simulink model "simulation_upgrade"  (R2024b)
settings: Solver=ode1be  StartTime=0.0  StopTime=10  FixedStep=0.001  RelTol=1e-3
model workspace (MAT data in the model file):
  AMP = 1
  FREQ = 1
  i_abc = 1
values from neighbouring files (symbols this model uses):
  v_WLTP = [0 0 0 0 0 0 0 0 0 0 0 0 ... (180001 elements, 1x180001)]    [v_WLTP.mat]
undefined symbols (not defined in the file or in its folder): A, a_sig, b_sig, C1, C2, C3, Cd, CG_z, downshift, Drive_wheel, Driveshaft, f_blend, f_OVD, fo, front_seat_dist, fs, g, Gearbox, i, i_sig, Inclination, Inertia, Jr2, K, m, M_curve_1, M_curve_2, m_driver, M_N_1, M_N_2, mi_c, mi_s, Mode, N_clutch, n_curve_1, n_curve_2, n_driver, n_max_1, n_max_2, n_shift, n_surfaces, Pl, Planetary, r_eq_clutch, r_geom, r_wheel, rho, Shaft, shift_time, sigma0, sigma1, sigma2, slope_angle, Stage1, Stage2, Stage3, upshift, v0, vel_wind, vs ... (+5)
libraries: simulink x29, slpidlib x3
(part 7 of 9)

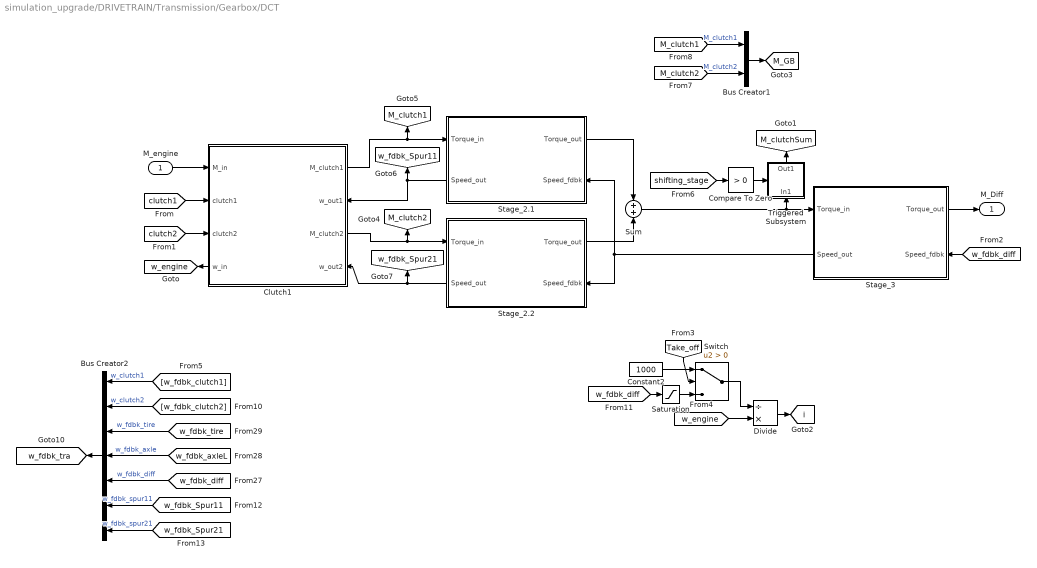
== system simulation_upgrade/DRIVETRAIN/Transmission/Gearbox/DCT ==
  M_engine : Inport
  Bus Creator1 : BusCreator  Inputs=2
  Bus Creator2 : BusCreator  Inputs=7
  Clutch1 : Subsystem
      settings: PortSchema="{\"entries\":[{\"content\":{\"sides\":[{\"content\":{\"connectorIds\":[\"In1\",\"In2\",\"In3\",\"Out3\"]},\"type\":\"ConnectorPlacement.EquallySpacedRectSide\",\"uuid\":\"d6060937-6a70-4d8f-85b8-f3c9c5d18f93\"},{\"content\":{\"connectorIds\":[\"Out1\",\"In4\",\"Out2\",\"In5\"],\"side\":\"RIGHT\"},\"type\":\"ConnectorPlacement.EquallySpacedRectSide\",\"uuid\":\"5f6b068d-fc68-4249-8013-bc3df4965ca3\"},{\"content\":{\"side\":\"TOP\"},\"type\":\"ConnectorPlacement.EquallySpacedRectSide\",\"uuid\":\"81b536de-881e-418d-8c02-7373631e1270\"}]},\"type\":\"ConnectorPlacement.EquallySpacedConnector\",\"uuid\":\"48438dfd-c2d0-4ff7-b57e-a1bd101206eb\"}],\"packageUris\":[\"http://schema.mathworks.com/mf0/Connector/R2020b\"],\"version\":\"1.0\"}"
      mask Display: image('images/clutch.jpg');
  Compare To Zero : simulink/Logic and Bit Operations/Compare To Zero  relop=>  OutDataTypeStr=boolean
  Constant2 : Constant  Value=1000
  Divide : Product  Inputs=/*
  Saturation : Saturate  UpperLimit=1000000  LowerLimit=1
  Stage_2.1 : Subsystem  Variant=on
      settings: PortSchema="{\"entries\":[{\"content\":{\"sides\":[{\"content\":{\"connectorIds\":[\"In1\",\"Out2\"]},\"type\":\"ConnectorPlacement.EquallySpacedRectSide\",\"uuid\":\"898fedf9-82f7-4bc2-bf05-880de36b191d\"},{\"content\":{\"connectorIds\":[\"Out1\",\"In2\"],\"side\":\"RIGHT\"},\"type\":\"ConnectorPlacement.EquallySpacedRectSide\",\"uuid\":\"50317b6c-245f-4bd1-a8cd-7a774957ae86\"},{\"content\":{\"side\":\"TOP\"},\"type\":\"ConnectorPlacement.EquallySpacedRectSide\",\"uuid\":\"ff1de2a1-7305-40d8-9e1f-fd0fa1e7d830\"}]},\"type\":\"ConnectorPlacement.EquallySpacedConnector\",\"uuid\":\"6ce82d73-f3da-4f59-9039-464a6ef3e9c5\"}],\"packageUris\":[\"http://schema.mathworks.com/mf0/Connector/R2020b\"],\"version\":\"1.0\"}"
      mask Display: image('images/branco.png');
  Stage_2.2 : Subsystem  Variant=on
      settings: PortSchema="{\"entries\":[{\"content\":{\"sides\":[{\"content\":{\"connectorIds\":[\"In1\",\"Out2\"]},\"type\":\"ConnectorPlacement.EquallySpacedRectSide\",\"uuid\":\"898fedf9-82f7-4bc2-bf05-880de36b191d\"},{\"content\":{\"connectorIds\":[\"Out1\",\"In2\"],\"side\":\"RIGHT\"},\"type\":\"ConnectorPlacement.EquallySpacedRectSide\",\"uuid\":\"50317b6c-245f-4bd1-a8cd-7a774957ae86\"},{\"content\":{\"side\":\"TOP\"},\"type\":\"ConnectorPlacement.EquallySpacedRectSide\",\"uuid\":\"ff1de2a1-7305-40d8-9e1f-fd0fa1e7d830\"}]},\"type\":\"ConnectorPlacement.EquallySpacedConnector\",\"uuid\":\"6ce82d73-f3da-4f59-9039-464a6ef3e9c5\"}],\"packageUris\":[\"http://schema.mathworks.com/mf0/Connector/R2020b\"],\"version\":\"1.0\"}"
      mask Display: image('images/branco.png');
  Stage_3 : Subsystem  Variant=on
      settings: PortSchema="{\"entries\":[{\"content\":{\"sides\":[{\"content\":{\"connectorIds\":[\"In1\",\"Out2\"]},\"type\":\"ConnectorPlacement.EquallySpacedRectSide\",\"uuid\":\"37b17ee8-4b62-4191-976c-22442f171034\"},{\"content\":{\"connectorIds\":[\"Out1\",\"In2\"],\"side\":\"RIGHT\"},\"type\":\"ConnectorPlacement.EquallySpacedRectSide\",\"uuid\":\"4dd88878-371f-49ed-bf90-7ed62e5325b4\"},{\"content\":{\"side\":\"TOP\"},\"type\":\"ConnectorPlacement.EquallySpacedRectSide\",\"uuid\":\"77efb153-e78e-4021-a08b-14751aa491e1\"}]},\"type\":\"ConnectorPlacement.EquallySpacedConnector\",\"uuid\":\"fa13ac12-58ae-4dfa-a455-8cf832864b15\"}],\"packageUris\":[\"http://schema.mathworks.com/mf0/Connector/R2020b\"],\"version\":\"1.0\"}"
      mask Display: image('images/branco.png');
  Sum : Sum  Inputs=+|+
  Switch : Switch  Criteria=u2 > Threshold  SaturateOnIntegerOverflow=off  InputSameDT=off
  Triggered Subsystem : Subsystem  TreatAsAtomicUnit=on
  M_Diff : Outport
  tag scope: M_GB=global, M_clutch1=global, M_clutch2=global, M_clutchSum=global, i=global, w_engine=global, w_fdbk_Spur11=global, w_fdbk_Spur21=global, w_fdbk_tra=global
  wires:
  Clutch1/1(M_clutch1) -> Stage_2.1/1(Torque_in), [M_clutch1]
  Bus Creator1/1 -> [M_GB]
  [w_fdbk_tire] -> Bus Creator2/3  "w_fdbk_tire"
  Switch/1 -> Divide/1
  [M_clutch1] -> Bus Creator1/1  "M_clutch1"
  [w_fdbk_clutch1] -> Bus Creator2/1  "w_clutch1"
  M_engine/1 -> Clutch1/1(M_in)
  Stage_3/2(Speed_out) -> Stage_2.1/2(Speed_fdbk), Stage_2.2/2(Speed_fdbk)
  [w_fdbk_diff] -> Saturation/1
  [w_fdbk_axleL] -> Bus Creator2/4  "w_fdbk_axle"
  [Take_off] -> Switch/2
  Bus Creator2/1 -> [w_fdbk_tra]
  [w_fdbk_diff] -> Stage_3/2(Speed_fdbk)
  Constant2/1 -> Switch/1
  Stage_3/1(Torque_out) -> M_Diff/1
  [w_fdbk_Spur21] -> Bus Creator2/7  "w_fdbk_spur21"
  Stage_2.1/2(Speed_out) -> Clutch1/4(w_out1), [w_fdbk_Spur11]
  Stage_2.1/1(Torque_out) -> Sum/1
  Stage_2.2/2(Speed_out) -> Clutch1/5(w_out2), [w_fdbk_Spur21]
  [w_fdbk_diff] -> Bus Creator2/5  "w_fdbk_diff"
  Divide/1 -> [i]
  Stage_2.2/1(Torque_out) -> Sum/2
  [w_fdbk_clutch2] -> Bus Creator2/2  "w_clutch2"
  [M_clutch2] -> Bus Creator1/2  "M_clutch2"
  [w_engine] -> Divide/2
  Saturation/1 -> Switch/3
  [w_fdbk_Spur11] -> Bus Creator2/6  "w_fdbk_spur11"
  Sum/1 -> Stage_3/1(Torque_in), Triggered Subsystem/1(In1)
  Clutch1/2(M_clutch2) -> [M_clutch2], Stage_2.2/1(Torque_in)
  Clutch1/3(w_in) -> [w_engine]
  [clutch1] -> Clutch1/2(clutch1)
  [clutch2] -> Clutch1/3(clutch2)
  Triggered Subsystem/1(Out1) -> [M_clutchSum]
  Compare To Zero/1 -> Triggered Subsystem/Trigger
  [shifting_stage] -> Compare To Zero/1

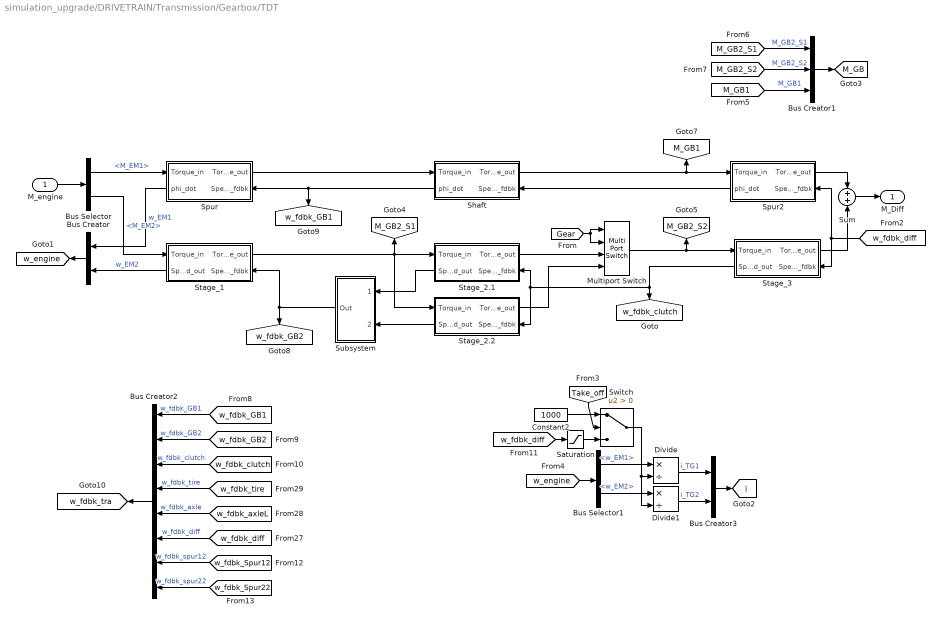
== system simulation_upgrade/DRIVETRAIN/Transmission/Gearbox/TDT ==
  M_engine : Inport
  Bus Creator : BusCreator  Inputs=2
  Bus Creator1 : BusCreator  Inputs=3
  Bus Creator2 : BusCreator  Inputs=8
  Bus Creator3 : BusCreator  Inputs=2
  Bus Selector : BusSelector  OutputSignals=M_EM1,M_EM2
  Bus Selector1 : BusSelector  OutputSignals=w_EM1,w_EM2
  Constant2 : Constant  Value=1000
  Divide : Product  Inputs=*/
  Divide1 : Product  Inputs=*/
  Multiport Switch : MultiPortSwitch  DataPortOrder=Zero-based contiguous  zeroidx=on  SaturateOnIntegerOverflow=off  InputSameDT=off
  Saturation : Saturate  UpperLimit=1000000  LowerLimit=1
  Shaft : Subsystem  mask{J=Shaft.J}
      mask prompts: J "Inertia_kgm^2"
      settings: PortSchema="{\"entries\":[{\"content\":{\"sides\":[{\"content\":{\"connectorIds\":[\"In1\",\"Out2\"]},\"type\":\"ConnectorPlacement.EquallySpacedRectSide\",\"uuid\":\"898fedf9-82f7-4bc2-bf05-880de36b191d\"},{\"content\":{\"connectorIds\":[\"Out1\",\"In2\"],\"side\":\"RIGHT\"},\"type\":\"ConnectorPlacement.EquallySpacedRectSide\",\"uuid\":\"50317b6c-245f-4bd1-a8cd-7a774957ae86\"},{\"content\":{\"side\":\"TOP\"},\"type\":\"ConnectorPlacement.EquallySpacedRectSide\",\"uuid\":\"ff1de2a1-7305-40d8-9e1f-fd0fa1e7d830\"}]},\"type\":\"ConnectorPlacement.EquallySpacedConnector\",\"uuid\":\"6ce82d73-f3da-4f59-9039-464a6ef3e9c5\"}],\"packageUris\":[\"http://schema.mathworks.com/mf0/Connector/R2020b\"],\"version\":\"1.0\"}"
  Spur : Subsystem  mask{i=Stage2.i1, J1=Stage2.Spur11.J, J2=Stage2.Spur12.J}
      mask prompts: i "Ratio"; J1 "Input_Gear_Inertia"; J2 "Output_Gear_Inertia"
      settings: PortSchema="{\"entries\":[{\"content\":{\"sides\":[{\"content\":{\"connectorIds\":[\"In1\",\"Out2\"]},\"type\":\"ConnectorPlacement.EquallySpacedRectSide\",\"uuid\":\"898fedf9-82f7-4bc2-bf05-880de36b191d\"},{\"content\":{\"connectorIds\":[\"Out1\",\"In2\"],\"side\":\"RIGHT\"},\"type\":\"ConnectorPlacement.EquallySpacedRectSide\",\"uuid\":\"50317b6c-245f-4bd1-a8cd-7a774957ae86\"},{\"content\":{\"side\":\"TOP\"},\"type\":\"ConnectorPlacement.EquallySpacedRectSide\",\"uuid\":\"ff1de2a1-7305-40d8-9e1f-fd0fa1e7d830\"}]},\"type\":\"ConnectorPlacement.EquallySpacedConnector\",\"uuid\":\"6ce82d73-f3da-4f59-9039-464a6ef3e9c5\"}],\"packageUris\":[\"http://schema.mathworks.com/mf0/Connector/R2020b\"],\"version\":\"1.0\"}"
  Spur2 : Subsystem  mask{i=Stage2.i1, J1=Stage2.Spur11.J, J2=Stage2.Spur12.J}
      mask prompts: i "Ratio"; J1 "Input_Gear_Inertia"; J2 "Output_Gear_Inertia"
      settings: PortSchema="{\"entries\":[{\"content\":{\"sides\":[{\"content\":{\"connectorIds\":[\"In1\",\"Out2\"]},\"type\":\"ConnectorPlacement.EquallySpacedRectSide\",\"uuid\":\"898fedf9-82f7-4bc2-bf05-880de36b191d\"},{\"content\":{\"connectorIds\":[\"Out1\",\"In2\"],\"side\":\"RIGHT\"},\"type\":\"ConnectorPlacement.EquallySpacedRectSide\",\"uuid\":\"50317b6c-245f-4bd1-a8cd-7a774957ae86\"},{\"content\":{\"side\":\"TOP\"},\"type\":\"ConnectorPlacement.EquallySpacedRectSide\",\"uuid\":\"ff1de2a1-7305-40d8-9e1f-fd0fa1e7d830\"}]},\"type\":\"ConnectorPlacement.EquallySpacedConnector\",\"uuid\":\"6ce82d73-f3da-4f59-9039-464a6ef3e9c5\"}],\"packageUris\":[\"http://schema.mathworks.com/mf0/Connector/R2020b\"],\"version\":\"1.0\"}"
  Stage_1 : Subsystem  Variant=on
      settings: PortSchema="{\"entries\":[{\"content\":{\"sides\":[{\"content\":{\"connectorIds\":[\"In1\",\"Out2\"]},\"type\":\"ConnectorPlacement.EquallySpacedRectSide\",\"uuid\":\"898fedf9-82f7-4bc2-bf05-880de36b191d\"},{\"content\":{\"connectorIds\":[\"Out1\",\"In2\"],\"side\":\"RIGHT\"},\"type\":\"ConnectorPlacement.EquallySpacedRectSide\",\"uuid\":\"50317b6c-245f-4bd1-a8cd-7a774957ae86\"},{\"content\":{\"side\":\"TOP\"},\"type\":\"ConnectorPlacement.EquallySpacedRectSide\",\"uuid\":\"ff1de2a1-7305-40d8-9e1f-fd0fa1e7d830\"}]},\"type\":\"ConnectorPlacement.EquallySpacedConnector\",\"uuid\":\"6ce82d73-f3da-4f59-9039-464a6ef3e9c5\"}],\"packageUris\":[\"http://schema.mathworks.com/mf0/Connector/R2020b\"],\"version\":\"1.0\"}"
      mask Display: image('images/branco.png');
  Stage_2.1 : Subsystem  Variant=on
      settings: PortSchema="{\"entries\":[{\"content\":{\"sides\":[{\"content\":{\"connectorIds\":[\"In1\",\"Out2\"]},\"type\":\"ConnectorPlacement.EquallySpacedRectSide\",\"uuid\":\"898fedf9-82f7-4bc2-bf05-880de36b191d\"},{\"content\":{\"connectorIds\":[\"Out1\",\"In2\"],\"side\":\"RIGHT\"},\"type\":\"ConnectorPlacement.EquallySpacedRectSide\",\"uuid\":\"50317b6c-245f-4bd1-a8cd-7a774957ae86\"},{\"content\":{\"side\":\"TOP\"},\"type\":\"ConnectorPlacement.EquallySpacedRectSide\",\"uuid\":\"ff1de2a1-7305-40d8-9e1f-fd0fa1e7d830\"}]},\"type\":\"ConnectorPlacement.EquallySpacedConnector\",\"uuid\":\"6ce82d73-f3da-4f59-9039-464a6ef3e9c5\"}],\"packageUris\":[\"http://schema.mathworks.com/mf0/Connector/R2020b\"],\"version\":\"1.0\"}"
      mask Display: image('images/branco.png');
  Stage_2.2 : Subsystem  Variant=on
      settings: PortSchema="{\"entries\":[{\"content\":{\"sides\":[{\"content\":{\"connectorIds\":[\"In1\",\"Out2\"]},\"type\":\"ConnectorPlacement.EquallySpacedRectSide\",\"uuid\":\"898fedf9-82f7-4bc2-bf05-880de36b191d\"},{\"content\":{\"connectorIds\":[\"Out1\",\"In2\"],\"side\":\"RIGHT\"},\"type\":\"ConnectorPlacement.EquallySpacedRectSide\",\"uuid\":\"50317b6c-245f-4bd1-a8cd-7a774957ae86\"},{\"content\":{\"side\":\"TOP\"},\"type\":\"ConnectorPlacement.EquallySpacedRectSide\",\"uuid\":\"ff1de2a1-7305-40d8-9e1f-fd0fa1e7d830\"}]},\"type\":\"ConnectorPlacement.EquallySpacedConnector\",\"uuid\":\"6ce82d73-f3da-4f59-9039-464a6ef3e9c5\"}],\"packageUris\":[\"http://schema.mathworks.com/mf0/Connector/R2020b\"],\"version\":\"1.0\"}"
      mask Display: image('images/branco.png');
  Stage_3 : Subsystem  Variant=on
      settings: PortSchema="{\"entries\":[{\"content\":{\"sides\":[{\"content\":{\"connectorIds\":[\"In1\",\"Out2\"]},\"type\":\"ConnectorPlacement.EquallySpacedRectSide\",\"uuid\":\"898fedf9-82f7-4bc2-bf05-880de36b191d\"},{\"content\":{\"connectorIds\":[\"Out1\",\"In2\"],\"side\":\"RIGHT\"},\"type\":\"ConnectorPlacement.EquallySpacedRectSide\",\"uuid\":\"50317b6c-245f-4bd1-a8cd-7a774957ae86\"},{\"content\":{\"side\":\"TOP\"},\"type\":\"ConnectorPlacement.EquallySpacedRectSide\",\"uuid\":\"ff1de2a1-7305-40d8-9e1f-fd0fa1e7d830\"}]},\"type\":\"ConnectorPlacement.EquallySpacedConnector\",\"uuid\":\"6ce82d73-f3da-4f59-9039-464a6ef3e9c5\"}],\"packageUris\":[\"http://schema.mathworks.com/mf0/Connector/R2020b\"],\"version\":\"1.0\"}"
      mask Display: image('images/branco.png');
  Subsystem : Subsystem
      settings: PortSchema="{\"entries\":[{\"content\":{\"sides\":[{\"content\":{\"connectorIds\":[\"Out1\"]},\"type\":\"ConnectorPlacement.EquallySpacedRectSide\",\"uuid\":\"fb6fb521-24b4-42a9-962b-0690c95a6555\"},{\"content\":{\"connectorIds\":[\"In1\",\"In2\"],\"side\":\"RIGHT\"},\"type\":\"ConnectorPlacement.EquallySpacedRectSide\",\"uuid\":\"05ff3728-9142-4ede-8c02-c3816594f1d6\"},{\"content\":{\"side\":\"TOP\"},\"type\":\"ConnectorPlacement.EquallySpacedRectSide\",\"uuid\":\"6bf5bb06-bb76-41b4-800b-6d1bd3df4c7c\"}]},\"type\":\"ConnectorPlacement.EquallySpacedConnector\",\"uuid\":\"4f0648fe-100b-4dfa-b2f8-0696c3f6a986\"}],\"packageUris\":[\"http://schema.mathworks.com/mf0/Connector/R2020b\"],\"version\":\"1.0\"}"
  Sum : Sum  Inputs=+|+
  Switch : Switch  Criteria=u2 > Threshold  SaturateOnIntegerOverflow=off  InputSameDT=off
  M_Diff : Outport
  tag scope: M_GB1=global, M_GB2_S1=global, M_GB2_S2=global, M_GB=global, i=global, w_engine=global, w_fdbk_GB1=global, w_fdbk_GB2=global, w_fdbk_clutch=global, w_fdbk_tra=global
  wires:
  M_engine/1 -> Bus Selector/1
  [Gear] -> Multiport Switch/2, Multiport Switch/1
  Multiport Switch/1 -> [M_GB2_S2], Stage_3/1(Torque_in)
  Stage_2.1/1(Torque_out) -> Multiport Switch/3
  Stage_1/2(Speed_out) -> Bus Creator/2  "w_EM2"
  Stage_2.2/1(Torque_out) -> Multiport Switch/4
  Stage_3/1(Torque_out) -> Sum/2
  Stage_2.1/2(Speed_out) -> Subsystem/1(Spur 21)
  Subsystem/1(Out) -> [w_fdbk_GB2], Stage_1/2(Speed_fdbk)
  Stage_3/2(Speed_out) -> Stage_2.2/2(Speed_fdbk), Stage_2.1/2(Speed_fdbk), [w_fdbk_clutch]
  Stage_1/1(Torque_out) -> Stage_2.1/1(Torque_in), [M_GB2_S1], Stage_2.2/1(Torque_in)
  Stage_2.2/2(Speed_out) -> Subsystem/2(Spur22)
  Shaft/1(Torque_out) -> Spur2/1(Torque_in), [M_GB1]
  Spur/1(Torque_out) -> Shaft/1(Torque_in)
  Spur2/2(phi_dot) -> Shaft/2(Speed_fdbk)
  Spur2/1(Torque_out) -> Sum/1
  [w_fdbk_diff] -> Spur2/2(Speed_fdbk), Stage_3/2(Speed_fdbk)
  Shaft/2(phi_dot) -> Spur/2(Speed_fdbk), [w_fdbk_GB1]
  Spur/2(phi_dot) -> Bus Creator/1  "w_EM1"
  Sum/1 -> M_Diff/1
  Bus Selector/2 -> Stage_1/1(Torque_in)  "<M_EM2>"
  Bus Selector/1 -> Spur/1(Torque_in)  "<M_EM1>"
  Bus Creator/1 -> [w_engine]
  Bus Creator1/1 -> [M_GB]
  [M_GB2_S2] -> Bus Creator1/2  "M_GB2_S2"
  [M_GB1] -> Bus Creator1/3  "M_GB1"
  [M_GB2_S1] -> Bus Creator1/1  "M_GB2_S1"
  [w_fdbk_GB1] -> Bus Creator2/1  "w_fdbk_GB1"
  [w_fdbk_GB2] -> Bus Creator2/2  "w_fdbk_GB2"
  [w_fdbk_clutch] -> Bus Creator2/3  "w_fdbk_clutch"
  Bus Creator2/1 -> [w_fdbk_tra]
  [w_fdbk_tire] -> Bus Creator2/4  "w_fdbk_tire"
  [w_fdbk_axleL] -> Bus Creator2/5  "w_fdbk_axle"
  [w_fdbk_diff] -> Bus Creator2/6  "w_fdbk_diff"
  [w_engine] -> Bus Selector1/1
  Bus Selector1/1 -> Divide/1  "<w_EM1>"
  Bus Selector1/2 -> Divide1/1  "<w_EM2>"
  Switch/1 -> Divide1/2, Divide/2
  Divide/1 -> Bus Creator3/1  "i_TG1"
  Divide1/1 -> Bus Creator3/2  "i_TG2"
  [w_fdbk_diff] -> Saturation/1
  [Take_off] -> Switch/2
  Constant2/1 -> Switch/1
  Bus Creator3/1 -> [i]
  Saturation/1 -> Switch/3
  [w_fdbk_Spur12] -> Bus Creator2/7  "w_fdbk_spur12"
  [w_fdbk_Spur22] -> Bus Creator2/8  "w_fdbk_spur22"

== system simulation_upgrade/DRIVETRAIN/Transmission/Gearbox/e-CVT ==
  M_engine : Inport
  M_Diff : Outport
  wires:
  M_engine/1 -> M_Diff/1

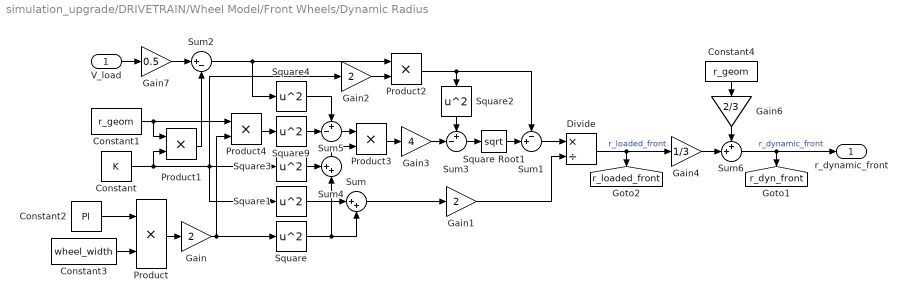
== system simulation_upgrade/DRIVETRAIN/Wheel Model/Front Wheels/Dynamic Radius ==
  V_load : Inport
  Constant : Constant  Value=K
  Constant1 : Constant  Value=r_geom
  Constant2 : Constant  Value=Pl
  Constant3 : Constant  Value=wheel_width
  Constant4 : Constant  Value=r_geom
  Divide : Product  Inputs=*/
  Gain : Gain  Gain=2
  Gain1 : Gain  Gain=2
  Gain2 : Gain  Gain=2
  Gain3 : Gain  Gain=4
  Gain4 : Gain  Gain=1/3
  Gain6 : Gain  Gain=2/3
  Gain7 : Gain  Gain=0.5
  Product{,1..4} (5 alike) : Product
  Square{,1..4,9} (6 alike) : Math  Operator=square
  Square Root1 : Sqrt
  Sum : Sum  Inputs=|++
  Sum1 : Sum  Inputs=-+|
  Sum2 : Sum  Inputs=|+-
  Sum3 : Sum  Inputs=+-|
  Sum4 : Sum  Inputs=++|
  Sum5 : Sum  Inputs=+-|
  Sum6 : Sum  Inputs=++|
  r_dynamic_front : Outport
  tag scope: r_dyn_front=global, r_loaded_front=global
  wires:
  Square1/1 -> Sum/1
  Divide/1 -> Gain4/1, [r_loaded_front]  "r_loaded_front"
  Square3/1 -> Sum4/1
  Sum/1 -> Gain1/1
  Sum1/1 -> Divide/1
  Constant/1 -> Product1/2, Square3/1, Gain2/1, Square1/1
  Constant3/1 -> Product/2
  Product1/1 -> Sum2/2
  Square Root1/1 -> Sum1/2
  Gain3/1 -> Sum3/2
  Gain/1 -> Product4/2, Square/1
  Constant2/1 -> Product/1
  Sum5/1 -> Product3/1
  Product3/1 -> Gain3/1
  Gain1/1 -> Divide/2
  Constant1/1 -> Product4/1, Product1/1
  Square9/1 -> Sum5/2
  Square/1 -> Sum4/2, Sum/2
  Sum4/1 -> Product3/2
  Sum3/1 -> Square Root1/1
  Square4/1 -> Sum5/1
  Sum2/1 -> Square4/1, Product2/1
  Product4/1 -> Square9/1
  Product/1 -> Gain/1
  Square2/1 -> Sum3/1
  Gain4/1 -> Sum6/2
  Gain6/1 -> Sum6/1
  Gain7/1 -> Sum2/1
  Constant4/1 -> Gain6/1
  Gain2/1 -> Product2/2
  Sum6/1 -> r_dynamic_front/1, [r_dyn_front]  "r_dynamic_front"
  Product2/1 -> Square2/1, Sum1/1
  V_load/1 -> Gain7/1

== system simulation_upgrade/DRIVETRAIN/Wheel Model/Front Wheels/Wheel Torque ==
  M_tra : Inport
  M_break : Inport  Port=2
  Bus Selector1 : BusSelector  OutputSignals=M_axleL,M_axleR
  Constant5 : Constant  Value=Drive_wheel
  Gain9 : Gain  Gain=0.5
  Multiport Switch : MultiPortSwitch  DataPortOrder=Zero-based contiguous  zeroidx=on  SaturateOnIntegerOverflow=off  InputSameDT=off
  Sum3 : Sum  Inputs=++|
  Sum4 : Sum  Inputs=++|
  Sum8 : Sum  Inputs=+|+
  M_front_wheels : Outport
  tag scope: M_front_wheels=global
  wires:
  Multiport Switch/1 -> M_front_wheels/1, [M_front_wheels]  "M_front_wheels"
  Bus Selector1/1 -> Sum8/1  "<M_axleL>"
  Constant5/1 -> Multiport Switch/1
  Gain9/1 -> Sum3/2
  M_break/1 -> Sum4/1, Sum3/1, Multiport Switch/2
  Bus Selector1/2 -> Sum8/2  "<M_axleR>"
  M_tra/1 -> Bus Selector1/1
  Sum8/1 -> Sum4/2, Gain9/1
  Sum3/1 -> Multiport Switch/4
  Sum4/1 -> Multiport Switch/3

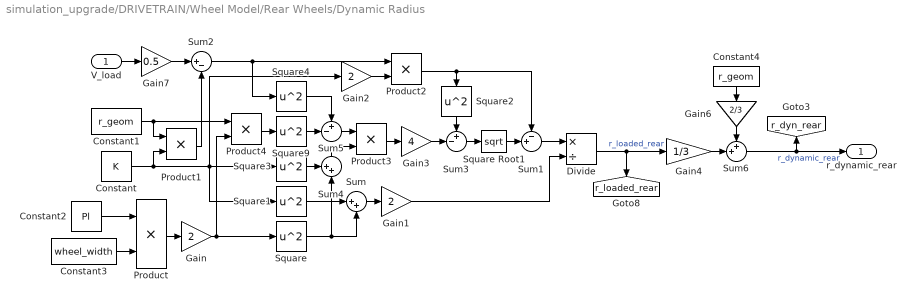
== system simulation_upgrade/DRIVETRAIN/Wheel Model/Rear Wheels/Dynamic Radius ==
  V_load : Inport
  Constant : Constant  Value=K
  Constant1 : Constant  Value=r_geom
  Constant2 : Constant  Value=Pl
  Constant3 : Constant  Value=wheel_width
  Constant4 : Constant  Value=r_geom
  Divide : Product  Inputs=*/
  Gain : Gain  Gain=2
  Gain1 : Gain  Gain=2
  Gain2 : Gain  Gain=2
  Gain3 : Gain  Gain=4
  Gain4 : Gain  Gain=1/3
  Gain6 : Gain  Gain=2/3
  Gain7 : Gain  Gain=0.5
  Product{,1..4} (5 alike) : Product
  Square{,1..4,9} (6 alike) : Math  Operator=square
  Square Root1 : Sqrt
  Sum : Sum  Inputs=|++
  Sum1 : Sum  Inputs=-+|
  Sum2 : Sum  Inputs=|+-
  Sum3 : Sum  Inputs=+-|
  Sum4 : Sum  Inputs=++|
  Sum5 : Sum  Inputs=+-|
  Sum6 : Sum  Inputs=++|
  r_dynamic_rear : Outport
  tag scope: r_dyn_rear=global, r_loaded_rear=global
  wires:
  Sum1/1 -> Divide/1
  Gain1/1 -> Divide/2
  Constant/1 -> Square1/1, Gain2/1, Square3/1, Product1/2
  Sum4/1 -> Product3/2
  Product2/1 -> Sum1/1, Square2/1
  Product1/1 -> Sum2/2
  Constant3/1 -> Product/2
  Square4/1 -> Sum5/1
  Product4/1 -> Square9/1
  Constant4/1 -> Gain6/1
  Gain4/1 -> Sum6/2
  Square1/1 -> Sum/1
  Square Root1/1 -> Sum1/2
  Gain/1 -> Square/1, Product4/2
  Sum2/1 -> Product2/1, Square4/1
  Gain3/1 -> Sum3/2
  Gain7/1 -> Sum2/1
  Sum3/1 -> Square Root1/1
  Gain6/1 -> Sum6/1
  Square9/1 -> Sum5/2
  Sum/1 -> Gain1/1
  Product3/1 -> Gain3/1
  Divide/1 -> [r_loaded_rear], Gain4/1  "r_loaded_rear"
  Gain2/1 -> Product2/2
  Square2/1 -> Sum3/1
  Constant1/1 -> Product1/1, Product4/1
  Sum6/1 -> r_dynamic_rear/1, [r_dyn_rear]  "r_dynamic_rear"
  V_load/1 -> Gain7/1
  Sum5/1 -> Product3/1
  Constant2/1 -> Product/1
  Product/1 -> Gain/1
  Square3/1 -> Sum4/1
  Square/1 -> Sum/2, Sum4/2

== system simulation_upgrade/DRIVETRAIN/Wheel Model/Rear Wheels/Wheel Torque ==
  M_tra : Inport
  M_break : Inport  Port=2
  Bus Selector1 : BusSelector  OutputSignals=M_axleL,M_axleR
  Constant5 : Constant  Value=Drive_wheel
  Gain : Gain  Gain=0.5
  Multiport Switch : MultiPortSwitch  DataPortOrder=Zero-based contiguous  zeroidx=on  SaturateOnIntegerOverflow=off  InputSameDT=off
  Sum : Sum  Inputs=|++
  Sum1 : Sum  Inputs=++|
  Sum8 : Sum  Inputs=+|+
  M_rear_wheels : Outport
  tag scope: M_rear_wheels=global
  wires:
  Multiport Switch/1 -> [M_rear_wheels], M_rear_wheels/1  "M_rear_wheels"
  Sum8/1 -> Gain/1, Sum/1
  Sum/1 -> Multiport Switch/2
  M_break/1 -> Sum/2, Sum1/1, Multiport Switch/3
  Bus Selector1/1 -> Sum8/1  "<M_axleL>"
  Bus Selector1/2 -> Sum8/2  "<M_axleR>"
  Constant5/1 -> Multiport Switch/1
  M_tra/1 -> Bus Selector1/1
  Gain/1 -> Sum1/2
  Sum1/1 -> Multiport Switch/4

== system simulation_upgrade/PANEL/Pretty shot/Transmission /Variant Subsystem ==
  note: 1) Add Subsystem or Model blocks as valid variant choices.
      | 2) You cannot connect blocks at this level. At simulation, connectivity is automatically
      | determined, based on the active variant and port name matching.
  " " : Inport
  Automated Manual Transmission : Subsystem  VariantControl=Gearbox == 2
      settings: PortSchema="{\"entries\":[{\"content\":{\"sides\":[{\"content\":{},\"type\":\"ConnectorPlacement.EquallySpacedRectSide\",\"uuid\":\"ed31482c-64ed-45d3-9038-ec800f8e1e41\"},{\"content\":{\"side\":\"RIGHT\"},\"type\":\"ConnectorPlacement.EquallySpacedRectSide\",\"uuid\":\"70c1b3a7-b724-464e-92eb-4c05fba4e9de\"},{\"content\":{\"connectorIds\":[\"Out1\"],\"side\":\"TOP\"},\"type\":\"ConnectorPlacement.EquallySpacedRectSide\",\"uuid\":\"8a0a3563-6c9b-4f19-bc40-18b3d82a8f82\"},{\"content\":{\"connectorIds\":[\"In1\"],\"side\":\"BOTTOM\"},\"type\":\"ConnectorPlacement.EquallySpacedRectSide\",\"uuid\":\"18c84272-fbb1-4cca-bc44-020313c1a3f2\"}]},\"type\":\"ConnectorPlacement.EquallySpacedConnector\",\"uuid\":\"9111ba9c-9409-40ea-8d81-f0edd42beba5\"}],\"packageUris\":[\"http://schema.mathworks.com/mf0/Connector/R2020b\"],\"version\":\"1.0\"}"
      mask Display: image('images/clutch.jpg');
  Automatic Transmission : Subsystem  VariantControl=Gearbox == 1
      settings: PortSchema="{\"entries\":[{\"content\":{\"sides\":[{\"content\":{},\"type\":\"ConnectorPlacement.EquallySpacedRectSide\",\"uuid\":\"ed31482c-64ed-45d3-9038-ec800f8e1e41\"},{\"content\":{\"side\":\"RIGHT\"},\"type\":\"ConnectorPlacement.EquallySpacedRectSide\",\"uuid\":\"70c1b3a7-b724-464e-92eb-4c05fba4e9de\"},{\"content\":{\"connectorIds\":[\"Out1\"],\"side\":\"TOP\"},\"type\":\"ConnectorPlacement.EquallySpacedRectSide\",\"uuid\":\"8a0a3563-6c9b-4f19-bc40-18b3d82a8f82\"},{\"content\":{\"connectorIds\":[\"In1\"],\"side\":\"BOTTOM\"},\"type\":\"ConnectorPlacement.EquallySpacedRectSide\",\"uuid\":\"e9fe4bba-d89d-42f2-a237-c1fc286bf7a9\"}]},\"type\":\"ConnectorPlacement.EquallySpacedConnector\",\"uuid\":\"9111ba9c-9409-40ea-8d81-f0edd42beba5\"}],\"packageUris\":[\"http://schema.mathworks.com/mf0/Connector/R2020b\"],\"version\":\"1.0\"}"
      mask Display: image('images/planetary.png');
  Twin Drive Transmission : Subsystem  VariantControl=Gearbox == 4
      settings: PortSchema="{\"entries\":[{\"content\":{\"sides\":[{\"content\":{},\"type\":\"ConnectorPlacement.EquallySpacedRectSide\",\"uuid\":\"ed31482c-64ed-45d3-9038-ec800f8e1e41\"},{\"content\":{\"side\":\"RIGHT\"},\"type\":\"ConnectorPlacement.EquallySpacedRectSide\",\"uuid\":\"70c1b3a7-b724-464e-92eb-4c05fba4e9de\"},{\"content\":{\"connectorIds\":[\"Out1\"],\"side\":\"TOP\"},\"type\":\"ConnectorPlacement.EquallySpacedRectSide\",\"uuid\":\"8a0a3563-6c9b-4f19-bc40-18b3d82a8f82\"},{\"content\":{\"connectorIds\":[\"In1\"],\"side\":\"BOTTOM\"},\"type\":\"ConnectorPlacement.EquallySpacedRectSide\",\"uuid\":\"38919f44-3f9f-4b3c-a934-63b0fa3950e5\"}]},\"type\":\"ConnectorPlacement.EquallySpacedConnector\",\"uuid\":\"9111ba9c-9409-40ea-8d81-f0edd42beba5\"}],\"packageUris\":[\"http://schema.mathworks.com/mf0/Connector/R2020b\"],\"version\":\"1.0\"}"
      mask Display: image('images/dog_clutch.png');
  "  " : Outport

== system simulation_upgrade/CONTROLS/Main Control Unit/AMT_MCU/Subsystem/Polynomial ==
  " " : Inport
  Constant : Constant  Value=5
  Constant1 : Constant  Value=4
  Constant2 : Constant  Value=3
  Constant3 : Constant  Value=C1
  Constant4 : Constant  Value=C2
  Constant5 : Constant  Value=C3
  Power : Math  Operator=pow
  Power1 : Math  Operator=pow
  Power2 : Math  Operator=pow
  Product1 : Product
  Product2 : Product
  Product3 : Product
  Sum1 : Sum  Inputs=+-+
  "  " : Outport
  wires:
  Product1/1 -> Sum1/1
  Constant4/1 -> Product2/2
  Constant5/1 -> Product3/2
  Constant2/1 -> Power2/2
  Constant1/1 -> Power/2
  Power/1 -> Product2/1
  Power1/1 -> Product1/1
  Product3/1 -> Sum1/3
  " "/1 -> Power2/1, Power1/1, Power/1
  Constant/1 -> Power1/2
  Product2/1 -> Sum1/2
  Power2/1 -> Product3/1
  Constant3/1 -> Product1/2
  Sum1/1 -> "  "/1

== system simulation_upgrade/CONTROLS/Main Control Unit/AMT_MCU/Subsystem/Sigmoid ==
  " " : Inport
  Constant6 : Constant
  Divide : Product  Inputs=*/
  Exp : Math
  Gain : Gain  Gain=a_sig
  Gain1 : Gain  Gain=b_sig
  Gain2 : Gain  Gain=1.003
  Sum3 : Sum  Inputs=++|
  Sum4 : Sum  Inputs=++|
  "  " : Outport
  wires:
  Exp/1 -> Sum3/2
  Sum4/1 -> Gain1/1
  Gain/1 -> Sum4/1
  Gain1/1 -> Exp/1
  Gain2/1 -> Divide/1
  Sum3/1 -> Divide/2
  Constant6/1 -> Sum3/1, Gain2/1, Gain/1
  " "/1 -> Sum4/2
  Divide/1 -> "  "/1

== system simulation_upgrade/CONTROLS/Main Control Unit/AMT_MCU/Subsystem/signal_register ==
  signal : Inport
  Trigger : TriggerPort  TriggerType=either  VariantControl=(inherit)  InitialTriggerSignalState=zero  PortDimensions=1
  Memory : Memory  InitialCondition=1  InheritSampleTime=on
  Subtract : Sum  Inputs=+-
  previous_value : Outport
  difference : Outport  Port=2
  wires:
  Subtract/1 -> difference/1
  Memory/1 -> Subtract/2, previous_value/1
  signal/1 -> Subtract/1, Memory/1

== system simulation_upgrade/CONTROLS/Main Control Unit/AMT_MCU/Subsystem/time_register ==
  t : Inport
  Trigger : TriggerPort  TriggerType=either  VariantControl=(inherit)  InitialTriggerSignalState=zero  PortDimensions=1
  t0 : Outport
  wires:
  t/1 -> t0/1

== system simulation_upgrade/CONTROLS/Main Control Unit/AT_MCU/Clutch_Profile/polynomial_s_response ==
  clutch1set : Inport
  Clock : Clock
  Constant : Constant  Value=5
  Constant1 : Constant  Value=4
  Constant2 : Constant  Value=3
  Constant3 : Constant  Value=C1
  Constant4 : Constant  Value=C2
  Constant5 : Constant  Value=C3
  Power : Math  Operator=pow
  Power1 : Math  Operator=pow
  Power2 : Math  Operator=pow
  Product{,1..3} (4 alike) : Product
  Saturation1 : Saturate  UpperLimit=1  LowerLimit=0
  Scope{1..4} (4 alike) : Scope
  Sum : Sum  Inputs=|-+
  Sum1 : Sum  Inputs=+-+
  Sum2 : Sum  Inputs=++|
  Transport Delay : TransportDelay  DelayTime=0.01
  signal_register : Subsystem
  time_register : Subsystem
  Out1 : Outport
  wires:
  clutch1set/1 -> Scope3/1, time_register/Trigger, signal_register/1(signal), signal_register/Trigger
  time_register/1(t0) -> Sum/1, Scope2/1
  Product/1 -> Sum2/2
  Clock/1 -> Sum/2, time_register/1(t)
  signal_register/2(difference) -> Product/1
  signal_register/1(previous_value) -> Sum2/1
  Sum/1 -> Power/1, Power1/1, Power2/1
  Constant2/1 -> Power2/2
  Constant1/1 -> Power/2
  Constant/1 -> Power1/2
  Power1/1 -> Product1/1
  Power2/1 -> Product3/1
  Power/1 -> Product2/1
  Constant3/1 -> Product1/2
  Constant4/1 -> Product2/2
  Constant5/1 -> Product3/2
  Product2/1 -> Sum1/2
  Product1/1 -> Sum1/1
  Product3/1 -> Sum1/3
  Sum1/1 -> Product/2
  Sum2/1 -> Transport Delay/1, Scope1/1
  Transport Delay/1 -> Saturation1/1
  Saturation1/1 -> Out1/1, Scope4/1

== system simulation_upgrade/CONTROLS/Main Control Unit/AT_MCU/Clutch_Profile/polynomial_s_response1 ==
  clutch2set : Inport
  Clock : Clock
  Constant : Constant  Value=5
  Constant1 : Constant  Value=4
  Constant2 : Constant  Value=3
  Constant3 : Constant  Value=C1
  Constant4 : Constant  Value=C2
  Constant5 : Constant  Value=C3
  Power : Math  Operator=pow
  Power1 : Math  Operator=pow
  Power2 : Math  Operator=pow
  Product{,1..3} (4 alike) : Product
  Saturation1 : Saturate  UpperLimit=1  LowerLimit=0
  Scope{1..4} (4 alike) : Scope
  Sum : Sum  Inputs=|-+
  Sum1 : Sum  Inputs=+-+
  Sum2 : Sum  Inputs=++|
  Transport Delay : TransportDelay  DelayTime=0.01
  signal_register : Subsystem
  time_register : Subsystem
  Out1 : Outport
  wires:
  Saturation1/1 -> Scope4/1, Out1/1
  Transport Delay/1 -> Saturation1/1
  Sum2/1 -> Scope1/1, Transport Delay/1
  Sum1/1 -> Product/2
  Product3/1 -> Sum1/3
  Product1/1 -> Sum1/1
  Product2/1 -> Sum1/2
  Constant5/1 -> Product3/2
  Constant4/1 -> Product2/2
  Constant3/1 -> Product1/2
  Power/1 -> Product2/1
  Power2/1 -> Product3/1
  Power1/1 -> Product1/1
  Constant/1 -> Power1/2
  Constant1/1 -> Power/2
  Constant2/1 -> Power2/2
  Sum/1 -> Power2/1, Power1/1, Power/1
  signal_register/1(previous_value) -> Sum2/1
  signal_register/2(difference) -> Product/1
  Clock/1 -> time_register/1(t), Sum/2
  Product/1 -> Sum2/2
  time_register/1(t0) -> Scope2/1, Sum/1
  clutch2set/1 -> signal_register/Trigger, signal_register/1(signal), time_register/Trigger, Scope3/1

== system simulation_upgrade/CONTROLS/Main Control Unit/AT_MCU/Clutch_Profile/sigmoid_response ==
  clutch1set : Inport
  Clock : Clock
  Constant : Constant
  Divide : Product  Inputs=*/
  Exp : Math
  Gain : Gain  Gain=a_sig
  Gain1 : Gain  Gain=b_sig
  Gain2 : Gain  Gain=1.003
  Gain3 : Gain  Gain=0.0015
  Product : Product
  Saturation1 : Saturate  UpperLimit=1  LowerLimit=0
  Scope{1..4} (4 alike) : Scope
  Sum : Sum  Inputs=++|
  Sum1 : Sum  Inputs=++-
  Sum2 : Sum  Inputs=++-
  Transport Delay : TransportDelay  DelayTime=0.01
  signal_register : Subsystem
  time_register : Subsystem
  Out1 : Outport
  wires:
  Sum1/1 -> Gain1/1
  Sum/1 -> Divide/2
  clutch1set/1 -> time_register/Trigger, signal_register/1(signal), signal_register/Trigger
  Exp/1 -> Sum/2
  time_register/1(t0) -> Scope2/1, Sum1/2
  Constant/1 -> Gain/1, Gain2/1, Sum/1
  Product/1 -> Sum2/2
  Clock/1 -> time_register/1(t), Sum1/3
  Gain/1 -> Sum1/1
  Gain1/1 -> Exp/1
  signal_register/1(previous_value) -> Sum2/1
  Divide/1 -> Scope4/1, Product/2
  signal_register/2(difference) -> Gain3/1, Product/1
  Saturation1/1 -> Scope3/1, Out1/1
  Sum2/1 -> Transport Delay/1, Scope1/1
  Transport Delay/1 -> Saturation1/1
  Gain2/1 -> Divide/1
  Gain3/1 -> Sum2/3

== system simulation_upgrade/CONTROLS/Main Control Unit/AT_MCU/Clutch_Profile/sigmoid_response1 ==
  clutch2set : Inport
  Clock : Clock
  Constant : Constant
  Divide : Product  Inputs=*/
  Exp : Math
  Gain : Gain  Gain=a_sig
  Gain1 : Gain  Gain=b_sig
  Gain2 : Gain  Gain=1.003
  Gain3 : Gain  Gain=0.0015
  Product : Product
  Saturation1 : Saturate  UpperLimit=1  LowerLimit=0
  Scope{1..4} (4 alike) : Scope
  Sum : Sum  Inputs=++|
  Sum1 : Sum  Inputs=++-
  Sum2 : Sum  Inputs=++-
  Transport Delay : TransportDelay  DelayTime=0.01
  signal_register : Subsystem
  time_register : Subsystem
  Out1 : Outport
  wires:
  Gain3/1 -> Sum2/3
  Gain2/1 -> Divide/1
  Transport Delay/1 -> Saturation1/1
  Sum2/1 -> Scope1/1, Transport Delay/1
  Saturation1/1 -> Out1/1, Scope3/1
  signal_register/2(difference) -> Product/1, Gain3/1
  Divide/1 -> Product/2, Scope4/1
  signal_register/1(previous_value) -> Sum2/1
  Gain1/1 -> Exp/1
  Gain/1 -> Sum1/1
  Clock/1 -> Sum1/3, time_register/1(t)
  Product/1 -> Sum2/2
  Constant/1 -> Sum/1, Gain2/1, Gain/1
  time_register/1(t0) -> Sum1/2, Scope2/1
  Exp/1 -> Sum/2
  clutch2set/1 -> signal_register/Trigger, signal_register/1(signal), time_register/Trigger
  Sum/1 -> Divide/2
  Sum1/1 -> Gain1/1

== system simulation_upgrade/CONTROLS/Main Control Unit/AT_MCU/Shifting Impulses/downshift impulse ==
  Event : Inport
  Constant : Constant
  Constant1 : Constant  Value=0
  Switch : Switch  Criteria=u2 > Threshold  SaturateOnIntegerOverflow=off  InputSameDT=off
  Impulse : Outport
  wires:
  Event/1 -> Switch/2
  Constant/1 -> Switch/1
  Constant1/1 -> Switch/3
  Switch/1 -> Impulse/1

== system simulation_upgrade/CONTROLS/Main Control Unit/AT_MCU/Shifting Impulses/upshift impulse ==
  Event : Inport
  Constant : Constant
  Constant1 : Constant  Value=0
  Switch : Switch  Criteria=u2 > Threshold  SaturateOnIntegerOverflow=off  InputSameDT=off
  Impulse : Outport
  wires:
  Event/1 -> Switch/2
  Constant/1 -> Switch/1
  Constant1/1 -> Switch/3
  Switch/1 -> Impulse/1

== system simulation_upgrade/CONTROLS/Main Control Unit/DCT_MCU/Subsystem/Hyperbolic ==
  " " : Inport
  Constant1 : Constant  Value=-10
  Constant2 : Constant
  Constant3 : Constant  Value=2
  Constant6 : Constant  Value=shift_time/2
  Divide : Product  Inputs=/**
  Divide1 : Product  Inputs=*/
  Exp : Math
  Exp1 : Math
  Sum : Sum  Inputs=|+-
  Sum1 : Sum  Inputs=-+|
  "  " : Outport
  wires:
  Divide1/1 -> "  "/1
  " "/1 -> Divide/3
  Constant1/1 -> Divide/2, Exp/1
  Divide/1 -> Exp1/1
  Constant6/1 -> Divide/1
  Exp/1 -> Sum1/2
  Exp1/1 -> Sum/1
  Sum/1 -> Divide1/1
  Sum1/1 -> Divide1/2
  Constant2/1 -> Sum/2
  Constant3/1 -> Sum1/1

== system simulation_upgrade/CONTROLS/Main Control Unit/DCT_MCU/Subsystem/Polynomial ==
  " " : Inport
  Constant : Constant  Value=5
  Constant1 : Constant  Value=4
  Constant2 : Constant  Value=3
  Constant3 : Constant  Value=C1
  Constant4 : Constant  Value=C2
  Constant5 : Constant  Value=C3
  Power : Math  Operator=pow
  Power1 : Math  Operator=pow
  Power2 : Math  Operator=pow
  Product1 : Product
  Product2 : Product
  Product3 : Product
  Sum1 : Sum  Inputs=+-+
  "  " : Outport
  wires:
  Product1/1 -> Sum1/1
  Constant4/1 -> Product2/2
  Constant5/1 -> Product3/2
  Constant2/1 -> Power2/2
  Constant1/1 -> Power/2
  Power/1 -> Product2/1
  Power1/1 -> Product1/1
  Product3/1 -> Sum1/3
  " "/1 -> Power2/1, Power1/1, Power/1
  Constant/1 -> Power1/2
  Product2/1 -> Sum1/2
  Power2/1 -> Product3/1
  Constant3/1 -> Product1/2
  Sum1/1 -> "  "/1

== system simulation_upgrade/CONTROLS/Main Control Unit/DCT_MCU/Subsystem/Sigmoid ==
  " " : Inport
  Constant6 : Constant
  Divide : Product  Inputs=*/
  Exp : Math
  Gain : Gain  Gain=a_sig
  Gain1 : Gain  Gain=b_sig
  Gain2 : Gain  Gain=1.003
  Sum3 : Sum  Inputs=++|
  Sum4 : Sum  Inputs=++|
  "  " : Outport
  wires:
  Exp/1 -> Sum3/2
  Sum4/1 -> Gain1/1
  Gain/1 -> Sum4/1
  Gain1/1 -> Exp/1
  Gain2/1 -> Divide/1
  Sum3/1 -> Divide/2
  Constant6/1 -> Sum3/1, Gain2/1, Gain/1
  " "/1 -> Sum4/2
  Divide/1 -> "  "/1

== system simulation_upgrade/CONTROLS/Main Control Unit/DCT_MCU/Subsystem/signal_register ==
  signal : Inport
  Trigger : TriggerPort  TriggerType=either  VariantControl=(inherit)  InitialTriggerSignalState=zero  PortDimensions=1
  Memory : Memory  InitialCondition=1  InheritSampleTime=on
  Subtract : Sum  Inputs=+-
  previous_value : Outport
  difference : Outport  Port=2
  wires:
  Subtract/1 -> difference/1
  Memory/1 -> Subtract/2, previous_value/1
  signal/1 -> Subtract/1, Memory/1

== system simulation_upgrade/CONTROLS/Main Control Unit/DCT_MCU/Subsystem/time_register ==
  t : Inport
  Trigger : TriggerPort  TriggerType=either  VariantControl=(inherit)  InitialTriggerSignalState=zero  PortDimensions=1
  t0 : Outport
  wires:
  t/1 -> t0/1

== system simulation_upgrade/CONTROLS/Main Control Unit/DCT_MCU/Subsystem1/Hyperbolic ==
  " " : Inport
  Constant1 : Constant  Value=-6
  Constant2 : Constant
  Constant6 : Constant  Value=shift_time
  Divide : Product  Inputs=/**
  Divide1 : Product  Inputs=*/
  Exp : Math
  Exp1 : Math
  Sum : Sum  Inputs=|+-
  Sum1 : Sum  Inputs=-+|
  "  " : Outport
  wires:
  Divide1/1 -> "  "/1
  " "/1 -> Divide/3
  Constant1/1 -> Divide/2, Exp/1
  Divide/1 -> Exp1/1
  Constant6/1 -> Divide/1
  Exp/1 -> Sum1/2
  Exp1/1 -> Sum/1
  Sum/1 -> Divide1/1
  Sum1/1 -> Divide1/2
  Constant2/1 -> Sum1/1, Sum/2

== system simulation_upgrade/CONTROLS/Main Control Unit/DCT_MCU/Subsystem1/Polynomial ==
  " " : Inport
  Constant : Constant  Value=5
  Constant1 : Constant  Value=4
  Constant2 : Constant  Value=3
  Constant3 : Constant  Value=C1
  Constant4 : Constant  Value=C2
  Constant5 : Constant  Value=C3
  Power : Math  Operator=pow
  Power1 : Math  Operator=pow
  Power2 : Math  Operator=pow
  Product1 : Product
  Product2 : Product
  Product3 : Product
  Sum1 : Sum  Inputs=+-+
  "  " : Outport
  wires:
  Sum1/1 -> "  "/1
  Constant3/1 -> Product1/2
  Power2/1 -> Product3/1
  Product2/1 -> Sum1/2
  Constant/1 -> Power1/2
  " "/1 -> Power/1, Power1/1, Power2/1
  Product3/1 -> Sum1/3
  Power1/1 -> Product1/1
  Power/1 -> Product2/1
  Constant1/1 -> Power/2
  Constant2/1 -> Power2/2
  Constant5/1 -> Product3/2
  Constant4/1 -> Product2/2
  Product1/1 -> Sum1/1

== system simulation_upgrade/CONTROLS/Main Control Unit/DCT_MCU/Subsystem1/Sigmoid ==
  " " : Inport
  Constant6 : Constant
  Divide : Product  Inputs=*/
  Exp : Math
  Gain : Gain  Gain=a_sig
  Gain1 : Gain  Gain=b_sig
  Gain2 : Gain  Gain=1.003
  Sum3 : Sum  Inputs=++|
  Sum4 : Sum  Inputs=++|
  "  " : Outport
  wires:
  Divide/1 -> "  "/1
  " "/1 -> Sum4/2
  Constant6/1 -> Gain/1, Gain2/1, Sum3/1
  Sum3/1 -> Divide/2
  Gain2/1 -> Divide/1
  Gain1/1 -> Exp/1
  Gain/1 -> Sum4/1
  Sum4/1 -> Gain1/1
  Exp/1 -> Sum3/2

== system simulation_upgrade/CONTROLS/Main Control Unit/DCT_MCU/Subsystem1/signal_register ==
  signal : Inport
  Trigger : TriggerPort  TriggerType=either  VariantControl=(inherit)  InitialTriggerSignalState=zero  PortDimensions=1
  Memory : Memory  InheritSampleTime=on
  Subtract : Sum  Inputs=+-
  previous_value : Outport
  difference : Outport  Port=2
  wires:
  signal/1 -> Memory/1, Subtract/1
  Memory/1 -> previous_value/1, Subtract/2
  Subtract/1 -> difference/1

== system simulation_upgrade/CONTROLS/Main Control Unit/DCT_MCU/Subsystem1/time_register ==
  t : Inport
  Trigger : TriggerPort  TriggerType=either  VariantControl=(inherit)  InitialTriggerSignalState=zero  PortDimensions=1
  t0 : Outport
  wires:
  t/1 -> t0/1

== system simulation_upgrade/DRIVETRAIN/Transmission/Gearbox/AMT/Clutch ==
  M_in : Inport
  " " : Inport  Port=2
  w_out : Inport  Port=3
  "  " : InportShadow  Port=2
  "   " : InportShadow  Port=2
  Abs : Abs  SaturateOnIntegerOverflow=off
  Clutch1 : Subsystem
      settings: PortSchema="{\"entries\":[{\"content\":{\"sides\":[{\"content\":{\"connectorIds\":[\"In1\"]},\"type\":\"ConnectorPlacement.EquallySpacedRectSide\",\"uuid\":\"a26f5a32-9f9c-4306-b7a8-6355090a4a86\"},{\"content\":{\"connectorIds\":[\"Out1\"],\"side\":\"RIGHT\"},\"type\":\"ConnectorPlacement.EquallySpacedRectSide\",\"uuid\":\"4fa489e2-cd1d-4a36-b0cb-261100046200\"},{\"content\":{\"connectorIds\":[\"In2\"],\"side\":\"TOP\"},\"type\":\"ConnectorPlacement.EquallySpacedRectSide\",\"uuid\":\"0e05a540-d6e3-4351-9a32-83f6c32571ff\"}]},\"type\":\"ConnectorPlacement.EquallySpacedConnector\",\"uuid\":\"492e0439-728a-4999-b29b-e2639b0e762e\"}],\"packageUris\":[\"http://schema.mathworks.com/mf0/Connector/R2020b\"],\"version\":\"1.0\"}"
  Compare To Constant2 : simulink/Logic and Bit Operations/Compare To Constant  relop===  const=0  OutDataTypeStr=boolean
  Constant2 : Constant  Value=N_clutch*mi_s*r_eq_clutch*n_surfaces
  Constant3 : Constant  Value=Shaft.J
  Delay : Delay  DelayLength=1  InputProcessing=Columns as channels (frame based)
  Delay1 : Delay  DelayLength=1  InputProcessing=Columns as channels (frame based)
  Divide : Product  Inputs=*/
  Gain : Gain  Gain=Stage2.Spur21.J
  Gain1 : Gain  Gain=20000
  Gain8 : Gain  Gain=i.S1
  Integrator2 : Integrator  ExternalReset=either  InitialConditionSource=external
  Integrator3 : Integrator  ExternalReset=either  InitialConditionSource=external
  Multiport Switch : MultiPortSwitch  DataPortOrder=Zero-based contiguous  zeroidx=on  SaturateOnIntegerOverflow=off  InputSameDT=off
  Scope1 : Scope  NumInputPorts=3
  Scope2 : Scope  NumInputPorts=3
  Scope5 : Scope  NumInputPorts=4
  Sum : Sum  Inputs=|++
  Sum1 : Sum  Inputs=|+-
  Sum3 : Sum  Inputs=|+-
  Switch1 : Switch  Criteria=u2 > Threshold  SaturateOnIntegerOverflow=off  InputSameDT=off
  M_clutch : Outport
  w_in : Outport  Port=2
  tag scope: w_clutch=global
  wires:
  Constant2/1 -> Scope1/3
  [Gear] -> Multiport Switch/1
  Multiport Switch/1 -> w_in/1, Sum3/1, Scope2/3  "w_in"
  Sum3/1 -> Clutch1/1(delta_w), Scope2/1  "delta_w1"
  Sum/1 -> Divide/2
  M_in/1 -> Scope1/2, Sum1/1
  Constant3/1 -> Sum/2
  w_out/1 -> Multiport Switch/2, Scope2/2, Sum3/2
  " "/1 -> Gain/1
  Gain/1 -> Abs/1
  Abs/1 -> Sum/1
  Clutch1/1(M_clutch) -> Sum1/2, Scope1/1, M_clutch/1
  Sum1/1 -> Divide/1
  Divide/1 -> Integrator3/1
  Switch1/1 -> Scope5/4, Multiport Switch/4, Multiport Switch/3, [w_clutch], Delay/1
  Gain8/1 -> Integrator2/1
  Integrator2/1 -> Integrator3/3, Switch1/1, Scope5/2  "fdfw"
  [w_dot] -> Gain8/1
  Compare To Constant2/1 -> Integrator3/2, Integrator2/2, Switch1/2, Gain1/1
  Gain1/1 -> Scope5/1  "signal"
  Delay/1 -> Integrator2/3
  Integrator3/1 -> Switch1/3, Scope5/3  "fdbk"
  "  "/1 -> Delay1/1
  Delay1/1 -> Compare To Constant2/1
  "   "/1 -> Clutch1/2(" ")

== system simulation_upgrade/DRIVETRAIN/Transmission/Gearbox/AMT/Stage_1 ==
  note: 1) Add Subsystem or Model blocks as valid variant choices.
      | 2) You cannot connect blocks at this level. At simulation, connectivity is automatically
      | determined, based on the active variant and port name matching.
  Torque_in : Inport
  Speed_fdbk : Inport  Port=2
  Nothing : Subsystem  VariantControl=Stage1.Type == 0
  Spur : Subsystem  VariantControl=Stage1.Type == 1
  Torque_out : Outport
  Speed_out : Outport  Port=2

== system simulation_upgrade/DRIVETRAIN/Transmission/Gearbox/AMT/Stage_2.1 ==
  note: 1) Add Subsystem or Model blocks as valid variant choices.
      | 2) You cannot connect blocks at this level. At simulation, connectivity is automatically
      | determined, based on the active variant and port name matching.
  Torque_in : Inport
  Speed_fdbk : Inport  Port=2
  Nothing : Subsystem  VariantControl=Stage2.Type == 0
  Spur : Subsystem  VariantControl=Stage2.Type == 1
  Torque_out : Outport
  Speed_out : Outport  Port=2

== system simulation_upgrade/DRIVETRAIN/Transmission/Gearbox/AMT/Stage_2.2 ==
  note: 1) Add Subsystem or Model blocks as valid variant choices.
      | 2) You cannot connect blocks at this level. At simulation, connectivity is automatically
      | determined, based on the active variant and port name matching.
  Torque_in : Inport
  Speed_fdbk : Inport  Port=2
  Nothing : Subsystem  VariantControl=Stage2.Type == 0
  Spur : Subsystem  VariantControl=Stage2.Type == 1
  Torque_out : Outport
  Speed_out : Outport  Port=2

== system simulation_upgrade/DRIVETRAIN/Transmission/Gearbox/AMT/Stage_3 ==
  note: 1) Add Subsystem or Model blocks as valid variant choices.
      | 2) You cannot connect blocks at this level. At simulation, connectivity is automatically
      | determined, based on the active variant and port name matching.
  Torque_in : Inport
  Speed_fdbk : Inport  Port=2
  Nothing : Subsystem  VariantControl=Stage3.Type == 0
  Spur : Subsystem  VariantControl=Stage3.Type == 1
  Torque_out : Outport
  Speed_out : Outport  Port=2

== system simulation_upgrade/DRIVETRAIN/Transmission/Gearbox/AT/Non-Inertial_Planetary ==
  Torque_sun : Inport
  w_fdbk_carrier : Inport  Port=2
  Constant : Constant  Value=Zs*(Zs+Zr)
  Constant1 : Constant  Value=Zs*Zr
  Constant2 : Constant  Value=Zs+Zr
  Constant3 : Constant
  Divide : Product  Inputs=/*
  Product : Product
  Product1 : Product
  Product2 : Product  Inputs=3
  Square : Math  Operator=square
  Sum1 : Sum  Inputs=+-|
  Sum6 : Sum
  Torque_carrier : Outport
  w_fdbk_rotor : Outport  Port=2
  wires:
  Divide/1 -> Product/2, Product1/1
  w_fdbk_carrier/1 -> Product1/2
  Sum6/1 -> Divide/1
  Constant3/1 -> Sum1/1
  Product2/1 -> Sum6/1
  Constant1/1 -> Product2/3
  Torque_sun/1 -> Product/1
  Sum1/1 -> Product2/1
  Product1/1 -> w_fdbk_rotor/1
  Constant2/1 -> Square/1
  Square/1 -> Divide/2
  [clutch2] -> Sum1/2
  [clutch1] -> Product2/2
  Constant/1 -> Sum6/2
  Product/1 -> Torque_carrier/1

== system simulation_upgrade/DRIVETRAIN/Transmission/Gearbox/AT/Planetary1 ==
  note: Ts*ws+Tr*wr = Tc*wc
  ws : Inport
  Ts : Inport  Port=2
  Tr : Inport  Port=3
  wc : Inport  Port=4
  Ring clutch : Inport  Port=5
  Constant : Constant  Value=100000
  Derivative : Derivative
  Derivative1 : Derivative
  Derivative2 : Derivative
  Divide : Product  Inputs=*/
  Gain : Gain  Gain=Zs/Zr
  Gain1 : Gain  Gain=(Zr+Zs)/Zr
  Gain2 : Gain  Gain=Js
  Gain3 : Gain  Gain=Jc
  Gain4 : Gain  Gain=Jr
  Gain5 : Gain  Gain=0.5
  Product{,1,6..7} (4 alike) : Product
  Ring clutch1 : InportShadow  Port=5
  Sum : Sum  Inputs=|++
  Sum1 : Sum  Inputs=-+|
  Sum2 : Sum  Inputs=-+-
  Sum3 : Sum  Inputs=++|
  Sum4 : Sum  Inputs=-+|
  Switch : Switch  Criteria=u2 > Threshold  SaturateOnIntegerOverflow=off  InputSameDT=off
  Tc : Outport
  wr : Outport  Port=2
  tag scope: M_sun_P1=global
  wires:
  Divide/1 -> Sum2/2  "Tc"
  Sum/1 -> Divide/1  "Pc"
  Product/1 -> Sum/1
  Gain1/1 -> Sum1/2
  ws/1 -> Derivative2/1, Product/2, Gain/1  "ws"
  Product6/1 -> Sum/2  "Tr"
  Gain/1 -> Sum1/1
  Ring clutch/1 -> Product7/2
  Tr/1 -> Product6/2
  Sum1/1 -> Product7/1
  Product7/1 -> Derivative1/1, Product6/1, wr/1  "wr"
  Derivative2/1 -> Gain2/1
  Gain2/1 -> Sum2/1
  Derivative/1 -> Gain3/1
  Gain3/1 -> Sum3/1
  Sum3/1 -> Sum2/3
  Derivative1/1 -> Gain4/1
  Gain4/1 -> Sum3/2
  Sum2/1 -> Tc/1
  Switch/1 -> Gain1/1, Derivative/1, Divide/2  "wc"
  Ring clutch1/1 -> Product1/1
  Ts/1 -> Product1/2, Sum4/2
  Product1/1 -> Sum4/1
  Gain5/1 -> Product/1, [M_sun_P1]
  wc/1 -> Switch/1, Switch/2
  Constant/1 -> Switch/3
  Sum4/1 -> Gain5/1

== system simulation_upgrade/DRIVETRAIN/Transmission/Gearbox/AT/Planetary2 ==
  ws : Inport
  Ts : Inport  Port=2
  Tr : Inport  Port=3
  wc : Inport  Port=4
  Ring clutch : Inport  Port=5
  Constant : Constant  Value=100000
  Derivative : Derivative
  Derivative1 : Derivative
  Derivative2 : Derivative
  Divide : Product  Inputs=*/
  Gain : Gain  Gain=Zs/Zr
  Gain1 : Gain  Gain=(Zr+Zs)/Zr
  Gain2 : Gain  Gain=Js
  Gain3 : Gain  Gain=Jc
  Gain4 : Gain  Gain=Jr
  Gain6 : Gain  Gain=0.5
  Product{,1..3} (4 alike) : Product
  Ring clutch1 : InportShadow  Port=5
  Sum : Sum  Inputs=|++
  Sum1 : Sum  Inputs=-+|
  Sum2 : Sum  Inputs=-+-
  Sum3 : Sum  Inputs=++|
  Sum4 : Sum  Inputs=-+|
  Switch : Switch  Criteria=u2 > Threshold  SaturateOnIntegerOverflow=off  InputSameDT=off
  Tc : Outport
  wr : Outport  Port=2
  tag scope: M_sun_P2=global
  wires:
  Sum2/1 -> Tc/1  "Tc"
  Gain4/1 -> Sum3/2
  Derivative1/1 -> Gain4/1
  Sum3/1 -> Sum2/3
  Gain3/1 -> Sum3/1
  Derivative/1 -> Gain3/1
  Gain2/1 -> Sum2/1
  Derivative2/1 -> Gain2/1
  Sum1/1 -> Product2/1
  Tr/1 -> Product3/2  "Tr"
  Ring clutch/1 -> Product2/2
  Gain/1 -> Sum1/1
  Product3/1 -> Sum/2  "Tr"
  ws/1 -> Gain/1, Product/2, Derivative2/1  "ws"
  Gain1/1 -> Sum1/2
  Ts/1 -> Sum4/2, Product1/2
  Product/1 -> Sum/1
  Sum/1 -> Divide/1
  Divide/1 -> Sum2/2
  Switch/1 -> Divide/2, Derivative/1, Gain1/1
  Ring clutch1/1 -> Product1/1
  Product1/1 -> Gain6/1
  Sum4/1 -> Product/1, [M_sun_P2]  "Ts"
  Gain6/1 -> Sum4/1
  Product2/1 -> Product3/1, Derivative1/1, wr/1
  Constant/1 -> Switch/3
  wc/1 -> Switch/2, Switch/1

== system simulation_upgrade/DRIVETRAIN/Transmission/Gearbox/AT/Shaft ==
  Torque_in : Inport
  Speed_fdbk : Inport  Port=2
  Derivative : Derivative
  Gain3 : Gain  Gain=J
  Sum1 : Sum  Inputs=|+-
  Torque_out : Outport
  phi_dot : Outport  Port=2
  wires:
  Sum1/1 -> Torque_out/1
  Gain3/1 -> Sum1/2
  Torque_in/1 -> Sum1/1
  Speed_fdbk/1 -> phi_dot/1, Derivative/1
  Derivative/1 -> Gain3/1

== system simulation_upgrade/DRIVETRAIN/Transmission/Gearbox/AT/Stage_3 ==
  note: 1) Add Subsystem or Model blocks as valid variant choices.
      | 2) You cannot connect blocks at this level. At simulation, connectivity is automatically
      | determined, based on the active variant and port name matching.
  Torque_in : Inport
  Speed_fdbk : Inport  Port=2
  Nothing : Subsystem  VariantControl=Stage3.Type == 0
  Spur : Subsystem  VariantControl=Stage3.Type == 1
  Torque_out : Outport
  Speed_out : Outport  Port=2
